simulink model "bille_synthese_CDRE"  (R2019a)
settings: Solver=ode45  StartTime=0.0  StopTime=20  RelTol=1e-3  EnableMultiTasking=on
values from neighbouring files (symbols this model uses):
  Ai = 1    [BallOnBeam.m]
  Bi = 1    [BallOnBeam.m]
  C = [k1 0]    [BallOnBeam.m]
  Ci = 1    [BallOnBeam.m]
  Di = 0    [BallOnBeam.m]
  f = 7E-5    (= 7e-05)    [BallOnBeam.m]
  Fe = acker(Ae, Be, [exp(-Te/taudes), exp(-Te/taudes), exp(-Te/taudes)/20])    [BallOnBeam.m]
  J = 4.6E-5    (= 4.6e-05)    [BallOnBeam.m]
  k = 0.026    [BallOnBeam.m]
  k1 = 7    [BallOnBeam.m]
  k2 = 28.65    [BallOnBeam.m]
  k3 = 0.0159    [BallOnBeam.m]
  kb = 6.1    [BallOnBeam.m]
  ki = 1.6    [BallOnBeam.m]
  kp = nm*J*wndes^2/(k2*k*ki)    (= 27.0462934428)    [BallOnBeam.m]
  kpi = rm*tii*ki/taudesi    (= 1.6)    [BallOnBeam.m]
  kv = (2*xides*J*wndes - f)/(kp*ki*k*k3)    (= 0.093347474441)    [BallOnBeam.m]
  Ld = acker(Ad', Cd', [0.3, 0.3])'    [BallOnBeam.m]
  lm = 0.001    [BallOnBeam.m]
  nm = 960    [BallOnBeam.m]
  rm = 0.33    [BallOnBeam.m]
  Te = 0.2    [BallOnBeam.m]
  tii = 0.5*lm/rm    (= 0.00151515151515)    [BallOnBeam.m]
undefined symbols (not defined in the file or in its folder): Ad, Bd
settings Model: ExtModeTrigMode=oneshot  ExtModeArmWhenConnect=off  Creator=khennouh  LastModifiedBy=DELL
settings DataIOCC: SaveFormat=Array  SignalLoggingSaveFormat=ModelDataLogs  ReturnWorkspaceOutputs=off
settings OptimizationCC: BlockReduction=off  BooleanDataType=off
settings DebuggingCC: SaveWithParameterizedLinksMsg=none  UnderspecifiedInitializationDetection=Classic  MergeDetectMultiDrivingBlocksExec=none  SignalResolutionControl=TryResolveAllWithWarning  MultiTaskDSMMsg=warning  MultiTaskCondExecSysMsg=none  PregeneratedLibrarySubsystemCodeDiagnostic=none  ArithmeticOperatorsInVariantConditions=warning
settings HardwareCC: TargetUnknown=on
settings ModelReferenceCC: PropagateSignalLabelsOutOfModel=off
settings SFSimCC: SimUseLocalCustomCode=off
settings RTWCC: RTWUseLocalCustomCode=off
settings CodeAppCC: StateflowObjectComments=on
settings GRTTargetCC: TargetLangStandard=C89/C90 (ANSI)  CombineOutputUpdateFcns=off  GRTInterface=on

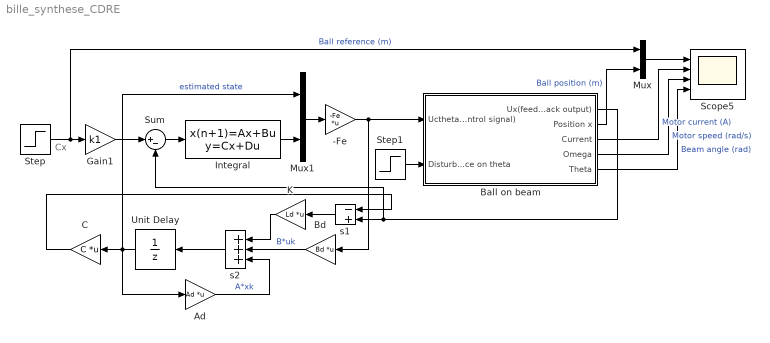
== system bille_synthese_CDRE ==
  note: Cx
  -Fe : Gain  Gain=-Fe  Multiplication=Matrix(K*u) (u vector)
  Ad : Gain  Gain=Ad  Multiplication=Matrix(K*u) (u vector)  SaturateOnIntegerOverflow=on  OutDataTypeStr=Inherit: Same as input  ParamDataTypeStr=Inherit: Same as input
  Ball on beam : Subsystem
  Bd : Gain  Gain=Bd  Multiplication=Matrix(K*u) (u vector)  SaturateOnIntegerOverflow=on  OutDataTypeStr=Inherit: Same as input  ParamDataTypeStr=Inherit: Same as input
  C : Gain  Gain=C  Multiplication=Matrix(K*u) (u vector)  SaturateOnIntegerOverflow=on  OutDataTypeStr=Inherit: Same as input  ParamDataTypeStr=Inherit: Same as input
  Gain1 : Gain  Gain=k1
  Integral : DiscreteStateSpace  A=Ai  B=Bi  C=Ci  D=Di  SampleTime=Te
  K : Gain  Gain=Ld  Multiplication=Matrix(K*u) (u vector)  SaturateOnIntegerOverflow=on  OutDataTypeStr=Inherit: Same as input  ParamDataTypeStr=Inherit: Same as input
  Mux : Mux  Inputs=2
  Mux1 : Mux  Inputs=2
  Scope5 : Scope  NumInputPorts=4
  Step : Step  After=0.1  SampleTime=0
  Step1 : Step  Time=10  After=1*pi/180  SampleTime=0
  Sum : Sum  Inputs=|+-
  Unit Delay : UnitDelay  SampleTime=Te  HasFrameUpgradeWarning=on
  s1 : Sum  Inputs=-+  SaturateOnIntegerOverflow=on  InputSameDT=on  OutDataTypeStr=Inherit: Same as first input
  s2 : Sum  Inputs=+++  SaturateOnIntegerOverflow=on  InputSameDT=on  OutDataTypeStr=Inherit: Same as first input
  wires:
  Step/1 -> Mux/1, Gain1/1  "Ball reference (m)"
  Mux/1 -> Scope5/1
  Gain1/1 -> Sum/1
  Step1/1 -> Ball on beam/2(Disturbance on theta)
  Ball on beam/2(Position x) -> Mux/2  "Ball position (m)"
  Ball on beam/3(Current) -> Scope5/2  "Motor current (A)"
  Ball on beam/4(" Omega") -> Scope5/3  "Motor speed (rad/s)"
  Ball on beam/5(" Theta") -> Scope5/4  "Beam angle (rad)"
  Ad/1 -> s2/3  "A*xk"
  s2/1 -> Unit Delay/1
  Bd/1 -> s2/2  "B*uk"
  s1/1 -> K/1
  K/1 -> s2/1
  C/1 -> s1/1
  -Fe/1 -> Bd/1, Ball on beam/1(Uctheta (control signal))
  Mux1/1 -> -Fe/1
  Sum/1 -> Integral/1
  Integral/1 -> Mux1/2
  Unit Delay/1 -> C/1, Ad/1, Mux1/1  "estimated state"
  Ball on beam/1(Ux(feedback output)) -> Sum/2, s1/2

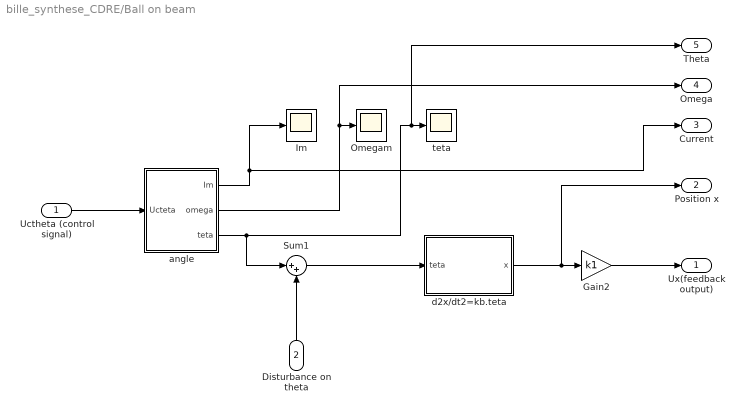
== system bille_synthese_CDRE/Ball on beam ==
  Uctheta (control signal) : Inport
  Disturbance on theta : Inport  Port=2
  Gain2 : Gain  Gain=k1
  Im : Scope
  Omegam : Scope
  Sum1 : Sum  Inputs=|++  SaturateOnIntegerOverflow=on  InputSameDT=on  OutDataTypeStr=Inherit: Same as first input
  angle : Subsystem
  "d2x/dt2=kb.teta " : Subsystem
  teta : Scope
  Ux(feedback output) : Outport
  Position x : Outport  Port=2
  Current : Outport  Port=3
  " Omega" : Outport  Port=4
  " Theta" : Outport  Port=5
  wires:
  angle/2(omega) -> " Omega"/1, Omegam/1
  Uctheta (control signal)/1 -> angle/1(Ucteta)
  Disturbance on theta/1 -> Sum1/2
  angle/3(teta) -> Sum1/1, " Theta"/1, teta/1
  angle/1(Im) -> Current/1, Im/1
  Gain2/1 -> Ux(feedback output)/1
  "d2x/dt2=kb.teta "/1(x) -> Position x/1, Gain2/1
  Sum1/1 -> "d2x/dt2=kb.teta "/1(teta)

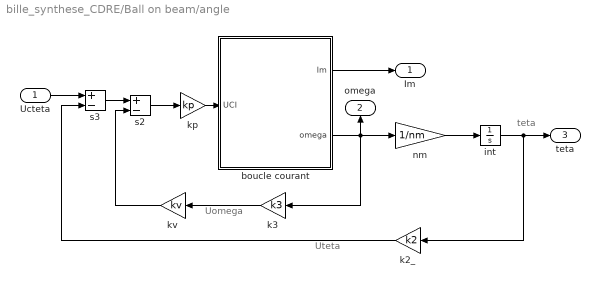
== system bille_synthese_CDRE/Ball on beam/angle ==
  note: Uomega
  note: teta
  note: Uteta
  Ucteta : Inport
  boucle courant : Subsystem
  int : Integrator
  k2_ : Gain  Gain=k2  SaturateOnIntegerOverflow=on  OutDataTypeStr=Inherit: Same as input  ParamDataTypeStr=Inherit: Same as input
  k3 : Gain  Gain=k3  SaturateOnIntegerOverflow=on  OutDataTypeStr=Inherit: Same as input  ParamDataTypeStr=Inherit: Same as input
  kp : Gain  Gain=kp  SaturateOnIntegerOverflow=on  OutDataTypeStr=Inherit: Same as input  ParamDataTypeStr=Inherit: Same as input
  kv : Gain  Gain=kv  SaturateOnIntegerOverflow=on  OutDataTypeStr=Inherit: Same as input  ParamDataTypeStr=Inherit: Same as input
  nm : Gain  Gain=1/nm  SaturateOnIntegerOverflow=on  OutDataTypeStr=Inherit: Same as input  ParamDataTypeStr=Inherit: Same as input
  s2 : Sum  Inputs=+-  SaturateOnIntegerOverflow=on  InputSameDT=on  OutDataTypeStr=Inherit: Same as first input
  s3 : Sum  Inputs=+-  SaturateOnIntegerOverflow=on  InputSameDT=on  OutDataTypeStr=Inherit: Same as first input
  Im : Outport
  omega : Outport  Port=2
  teta : Outport  Port=3
  wires:
  kp/1 -> boucle courant/1(UCI)
  s2/1 -> kp/1
  s3/1 -> s2/1
  nm/1 -> int/1
  boucle courant/2(omega) -> nm/1, k3/1, omega/1
  k3/1 -> kv/1
  kv/1 -> s2/2
  int/1 -> k2_/1, teta/1
  k2_/1 -> s3/2
  boucle courant/1(Im) -> Im/1
  Ucteta/1 -> s3/1

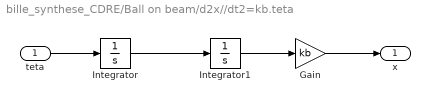
== system bille_synthese_CDRE/Ball on beam/d2x//dt2=kb.teta  ==
  teta : Inport
  Gain : Gain  Gain=kb
  Integrator : Integrator
  Integrator1 : Integrator
  x : Outport
  wires:
  Integrator/1 -> Integrator1/1
  teta/1 -> Integrator/1
  Integrator1/1 -> Gain/1
  Gain/1 -> x/1

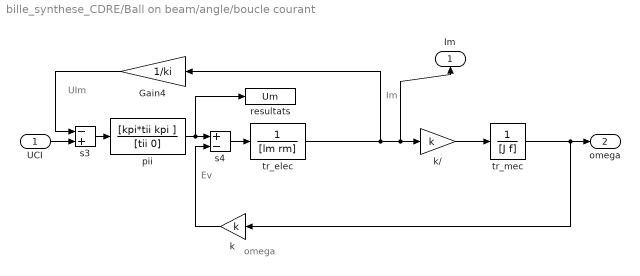
== system bille_synthese_CDRE/Ball on beam/angle/boucle courant ==
  note: Im
  note: Ev
  note: UIm
  note: omega
  UCI : Inport
  Gain4 : Gain  Gain=1/ki  SaturateOnIntegerOverflow=on  OutDataTypeStr=Inherit: Same as input  ParamDataTypeStr=Inherit: Same as input
  k : Gain  Gain=k  SaturateOnIntegerOverflow=on  OutDataTypeStr=Inherit: Same as input  ParamDataTypeStr=Inherit: Same as input
  "k/ " : Gain  Gain=k  SaturateOnIntegerOverflow=on  OutDataTypeStr=Inherit: Same as input  ParamDataTypeStr=Inherit: Same as input
  pii : TransferFcn  Numerator=[kpi*tii kpi ]  Denominator=[tii 0]
  resultats : ToWorkspace  VariableName=Um
      settings: MaxDataPoints=20000
  s3 : Sum  Inputs=-+  SaturateOnIntegerOverflow=on  InputSameDT=on  OutDataTypeStr=Inherit: Same as first input
  s4 : Sum  Inputs=+-  SaturateOnIntegerOverflow=on  InputSameDT=on  OutDataTypeStr=Inherit: Same as first input
  tr_elec : TransferFcn  Denominator=[lm rm]
  tr_mec : TransferFcn  Denominator=[J f]
  Im : Outport
  omega : Outport  Port=2
  wires:
  s4/1 -> tr_elec/1
  Gain4/1 -> s3/1
  s3/1 -> pii/1
  k/1 -> s4/2
  "k/ "/1 -> tr_mec/1
  tr_mec/1 -> k/1, omega/1
  UCI/1 -> s3/2
  pii/1 -> s4/1, resultats/1
  tr_elec/1 -> Gain4/1, "k/ "/1, Im/1
